simulink model "imcpendel4"  (R2021b)
settings: Solver=ode15s  StartTime=0.0  StopTime=1000  RelTol=1e-3
values from neighbouring files (symbols this model uses):
  A = double(A)    [Eindampfanlage.m]
  B = double(B)    [Eindampfanlage.m]
  C = double(C)    [Eindampfanlage.m]
  D = zeros(p,m)    [Eindampfanlage.m]
  uR1 = [214.13; 3.33+0.02; 65.40]    [Eindampfanlage.m]
  uR_offset = uR - uR_punkt_offset    [Eindampfanlage.m]
  x0 = [1; 25; 50]    [Eindampfanlage.m]
  xR = [1; 15; 70]    [Eindampfanlage.m]
undefined symbols (not defined in the file or in its folder): a, b, c, d
settings Model: Creator=mluser  LastModifiedBy=1star
settings DebuggingCC: UnconnectedInputMsg=none  UnconnectedOutputMsg=none  UnconnectedLineMsg=none
settings ModelReferenceCC: EnableRefExpFcnMdlSchedulingChecks=off
settings RTWCC: DLArmComputeVersion=20.02.1

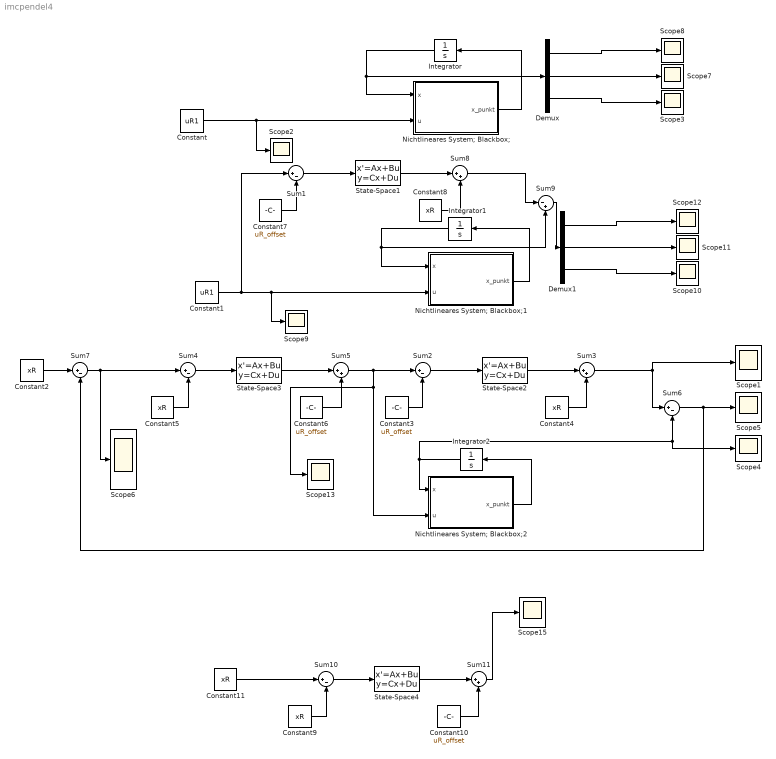
== system imcpendel4 ==
  Constant : Constant  Value=uR1
  Constant1 : Constant  Value=uR1
  Constant{3,6..7,10} (4 alike) : Constant  Value=uR_offset
  Constant{2,4..5,8..9,11} (6 alike) : Constant  Value=xR
  Demux : Demux  Outputs=3
  Demux1 : Demux  Outputs=3
  Integrator : Integrator  InitialCondition=x0
  Integrator1 : Integrator  InitialCondition=x0
  Integrator2 : Integrator  InitialCondition=x0
  Nichtlineares System; Blackbox; : MATLAB Function
  Nichtlineares System; Blackbox;1 : MATLAB Function
  Nichtlineares System; Blackbox;2 : MATLAB Function
  Scope{1..13,15} (14 alike) : Scope
  State-Space1 : StateSpace  A=A  B=B  C=C  D=D  InitialCondition=x0-xR
  State-Space2 : StateSpace  A=A  B=B  C=C  D=D  InitialCondition=x0-xR
  State-Space3 : StateSpace  A=a  B=b  C=c  D=d  InitialCondition=0  ParameterTunability=Optimized
  State-Space4 : StateSpace  A=a  B=b  C=c  D=d  InitialCondition=0  ParameterTunability=Optimized
  Sum{1..2,4,6..7,10} (6 alike) : Sum  Inputs=|+-
  Sum{3,5,8,11} (4 alike) : Sum  Inputs=|++
  Sum9 : Sum  Inputs=|-+
  wires:
  Nichtlineares System; Blackbox;/1(x_punkt) -> Integrator/1
  Integrator/1 -> Demux/1, Nichtlineares System; Blackbox;/1(x)
  Constant/1 -> Scope2/1, Nichtlineares System; Blackbox;/2(u)
  Sum2/1 -> State-Space2/1
  Constant3/1 -> Sum2/2
  State-Space2/1 -> Sum3/1
  Sum3/1 -> Sum6/1, Scope1/1
  Constant4/1 -> Sum3/2
  Constant6/1 -> Sum5/2
  State-Space3/1 -> Sum5/1
  Constant5/1 -> Sum4/2
  Sum4/1 -> State-Space3/1
  Nichtlineares System; Blackbox;2/1(x_punkt) -> Integrator2/1
  Integrator2/1 -> Nichtlineares System; Blackbox;2/1(x), Scope4/1, Sum6/2
  Sum5/1 -> Scope13/1, Nichtlineares System; Blackbox;2/2(u), Sum2/1
  Constant2/1 -> Sum7/1
  Sum7/1 -> Sum4/1, Scope6/1
  Demux/1 -> Scope8/1
  Demux/2 -> Scope7/1
  Demux/3 -> Scope3/1
  Demux1/2 -> Scope11/1
  Demux1/1 -> Scope12/1
  Demux1/3 -> Scope10/1
  Nichtlineares System; Blackbox;1/1(x_punkt) -> Integrator1/1
  Constant1/1 -> Scope9/1, Nichtlineares System; Blackbox;1/2(u), Sum1/1
  Sum8/1 -> Sum9/1
  Constant8/1 -> Sum8/2
  State-Space1/1 -> Sum8/1
  Sum1/1 -> State-Space1/1
  Integrator1/1 -> Sum9/2, Nichtlineares System; Blackbox;1/1(x)
  Constant7/1 -> Sum1/2
  Sum9/1 -> Demux1/1
  Sum6/1 -> Sum7/2, Scope5/1
  Constant11/1 -> Sum10/1
  State-Space4/1 -> Sum11/1
  Sum10/1 -> State-Space4/1
  Constant9/1 -> Sum10/2
  Constant10/1 -> Sum11/2
  Sum11/1 -> Scope15/1

== matlab function imcpendel4/Nichtlineares System; Blackbox; ==
  data: x input; x_punkt output; u input
function x_punkt = fcn(x, u)
a1 = 0.00751;
a2 = 0.00418;
a3 = 0.05;
a4 = 0.03755;
a5 = 0.02091;
a6 = 0.00315;

b1 = 0.00192;
b2 = 0.05;
b3 = 0.00959;
b4 = 0.1866;
b5 = 0.14;

k1 = 0.01061;
k2 = 2.5;
k3 = 6.84;
k4 = 2.5531;

x1_punkt = a1*x(3)+a2*x(2)-b1*u(1)-b2*u(2)-k1;
x2_punkt = -a3*x(2)*u(2)+k2;
x3_punkt = -a4*x(3)-a5*x(2)+b3*u(1)-(a6*x(3)+b4)*u(3)/(b5*u(3)+k3)+k4;

x_punkt = [x1_punkt;x2_punkt;x3_punkt];

== matlab function imcpendel4/Nichtlineares System; Blackbox;1 ==
  data: x input; x_punkt output; u input
function x_punkt = fcn(x, u)
a1 = 0.00751;
a2 = 0.00418;
a3 = 0.05;
a4 = 0.03755;
a5 = 0.02091;
a6 = 0.00315;

b1 = 0.00192;
b2 = 0.05;
b3 = 0.00959;
b4 = 0.1866;
b5 = 0.14;

k1 = 0.01061;
k2 = 2.5;
k3 = 6.84;
k4 = 2.5531;

x1_punkt = a1*x(3)+a2*x(2)-b1*u(1)-b2*u(2)-k1;
x2_punkt = -a3*x(2)*u(2)+k2;
x3_punkt = -a4*x(3)-a5*x(2)+b3*u(1)-(a6*x(3)+b4)*u(3)/(b5*u(3)+k3)+k4;

x_punkt = [x1_punkt;x2_punkt;x3_punkt];

== matlab function imcpendel4/Nichtlineares System; Blackbox;2 ==
  data: x input; x_punkt output; u input
function x_punkt = fcn(x, u)
a1 = 0.00751;
a2 = 0.00418;
a3 = 0.05;
a4 = 0.03755;
a5 = 0.02091;
a6 = 0.00315;

b1 = 0.00192;
b2 = 0.05;
b3 = 0.00959;
b4 = 0.1866;
b5 = 0.14;

k1 = 0.01061;
k2 = 2.5;
k3 = 6.84;
k4 = 2.5531;

x1_punkt = a1*x(3)+a2*x(2)-b1*u(1)-b2*u(2)-k1;
x2_punkt = -a3*x(2)*u(2)+k2;
x3_punkt = -a4*x(3)-a5*x(2)+b3*u(1)-(a6*x(3)+b4)*u(3)/(b5*u(3)+k3)+k4;

x_punkt = [x1_punkt;x2_punkt;x3_punkt];
